simulink model "BATTERY_PV_IMPLEMENTATION"  (R2024a)
settings: Solver=VariableStepAuto  StartTime=0.0  StopTime=0.23  RelTol=1e-3
values from neighbouring files (symbols this model uses):
  a = 1.3    [TEST.m]    (also in batter_y.m = -k_omega / J)
  beta = [0.0000, 0.0306, 0.0560, 0.0772, 0.0953, 0.1113, 0.1254, 0.1382,          0.1499, 0.1607, 0.1783, 0.2134, 0.2421, 0.2669, 0.2890, 0.3091,          0.3279, 0.3456, 0.3625, 0.3789]'    [batter_y.m]
  Cdc = 278e-3    (= 0.278)    [TEST.m]    (also in batter_y.m)
  Clink = 2 * (3 / 4) * (Pnom / Fnom * 2 / Vnom_dc^2)    (= 0.325520833333)    [batter_y.m]
  fg = 60    [TEST.m]    (also in batter_y.m)
  Fnom = 60    [batter_y.m]
  Gn = 1000    [TEST.m]    (also in batter_y.m)
  Ipv_n = Isc_n*(Rp+Rs)/Rp    (= 8.21426513558)    [TEST.m]    (also in batter_y.m)
  Isc_n = 8.21    [TEST.m]    (also in batter_y.m)
  k = 1.3806503e-23    [TEST.m]    (also in batter_y.m)
  k_I = a./(b.*tau_ref)    [batter_y.m]
  k_P = 5./(b.*tau_ref)    [batter_y.m]
  KI = 0.0032    [TEST.m]    (also in batter_y.m)
  Ki_C = Rc/tau_C    (= 0.768)    [TEST.m]    (also in batter_y.m)
  Ki_DC = omega_DC^2*Cdc    [TEST.m]    (also in batter_y.m)
  Ki_Ireg = 20    [batter_y.m]
  Ki_P = 1/(Ki_pq*tau_P)    [TEST.m]    (also in batter_y.m)
  Ki_PLL = Kp_PLL/tau_PLL    [TEST.m]    (also in batter_y.m)
  Kp_C = Lc/tau_C    (= 0.020372)    [TEST.m]    (also in batter_y.m)
  Kp_DC = 2*xi_DC*omega_DC*Cdc    [TEST.m]    (also in batter_y.m)
  Kp_Ireg = 0.3    [batter_y.m]
  Kp_P = tau_C/(Ki_pq*tau_P)    [TEST.m]    (also in batter_y.m)
  Kp_PLL = xi_PLL*2*omega_PLL/Vp    [TEST.m]    (also in batter_y.m)
  KV = -0.123    [TEST.m]    (also in batter_y.m)
  KVmp = Vmp_n/Voc_n    (= 0.799392097264)    [TEST.m]    (also in batter_y.m)
  Lc = 20.372e-6    (= 2.0372e-05)    [TEST.m]    (also in batter_y.m)
  Lchoke = 0.15    [batter_y.m]
  Ltot_pu = Lxf + Lchoke    (= 0.21)    [batter_y.m]
  Lxf = TotalLeakage    (= 0.06)    [batter_y.m]
  Np = 345    [TEST.m]    (also in batter_y.m)
  Ns = 45    [TEST.m]    (also in batter_y.m)
  Ns_cell = 54    [TEST.m]    (also in batter_y.m)
  Pnom = PnomkW*1e3    (= 500000)    [TEST.m]    (also in batter_y.m = 1500000)
  q = 1.6021764e-19    [TEST.m]    (also in batter_y.m)
  Rc = 0.768e-3    (= 0.000768)    [TEST.m]    (also in batter_y.m)
  Rchoke = 0.15 / 100    (= 0.0015)    [batter_y.m]
  Rp = 425.405    [TEST.m]    (also in batter_y.m)
  Rs = 0.221    [TEST.m]    (also in batter_y.m)
  Rtot_pu = Rxf + Rchoke    (= 0.0039)    [batter_y.m]
  Rxf = TotalLeakage / 25    (= 0.0024)    [batter_y.m]
  Tn = 25    [TEST.m]    (also in batter_y.m)
  Ts = 5e-5    (= 5e-05)    [TEST.m]    (also in batter_y.m)
  Ts_Control = 5e-5    (= 5e-05)    [TEST.m]    (also in batter_y.m)
  v = [11.2600, 11.5378, 11.8156, 12.0933, 12.3711, 12.6489, 12.9267,       13.2044, 13.4822, 13.7600, 14.2600, 15.4533, 16.6467, 17.8400,       19.0333, 20.2267, 21.4200, 22.6133, 23.8067, 25.0000]'    [batter_y.m]
  Vdc = 1200    [TEST.m]    (also in batter_y.m)
  Vnom_dc = 480    [batter_y.m]
  Vnom_prim = 2400    [batter_y.m]
  Vnom_sec = 0.85 * Vnom_dc / 2 / sqrt(2) * sqrt(3)    [batter_y.m]
  Voc_n = 32.9    [TEST.m]    (also in batter_y.m)
  Vp = Ug*sqrt(2)/sqrt(3)    [TEST.m]    (also in batter_y.m)
  Zbase = Vnom_sec^2 / Pnom    [batter_y.m]
undefined symbols (not defined in the file or in its folder): D1, Delta, Ion, Lithium, para_mdl
libraries: spsSeriesRLCBranchLib x25, slpidlib x11, spsThreePhaseSeriesRLCLoadLib x9, spsThreePhaseVIMeasurementLib x7, spsSeriesRLCLoadLib x5, spsGroundLib x5, spsThreePhaseTransformerTwoWindingsLib x5, spsabctodq0Lib x4, spsControlledVoltageSourceLib x3, spsPower3phInstantaneousLib x3, spsCurrentMeasurementLib x2, spsControlledCurrentSourceLib x2
(part 1 of 3)
settings Model: Creator=Dell  LastModifiedBy=Dell

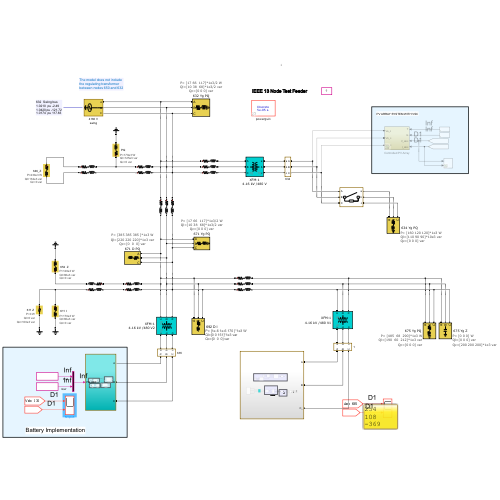
[thumbnail: Simulink's stored preview of the top-level diagram]
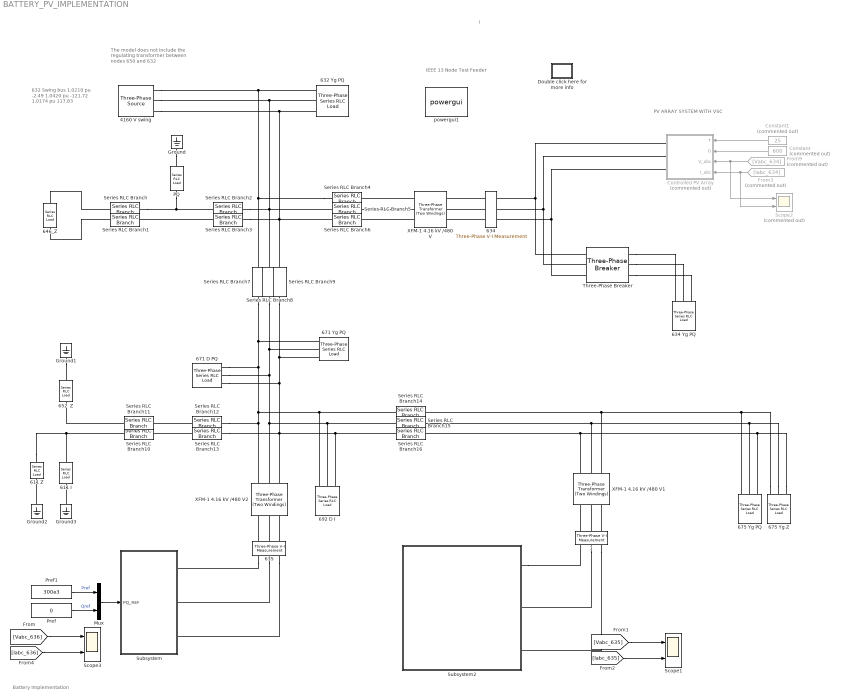
== system BATTERY_PV_IMPLEMENTATION ==
  note: Battery Implementation
  note: i
  note: PV ARRAY SYSTEM WITH VSC
  note: IEEE 13 Node Test Feeder
  note: The model does not include
      | the regulating transformer
      | between nodes 650 and 632
  note: 632 Swing bus
      | 1.0210 pu -2.49
      | 1.0420 pu -121.72
      | 1.0174 pu 117.83
  " 634 Yg PQ " : spsThreePhaseSeriesRLCLoadLib/Three-Phase Series RLC Load  LConnTagsString=A|B|C  Configuration=Y (grounded)  NominalVoltage=120e3  Vabc=[ 0.993805 1.0218 0.995862]*277.128  Vabcp=[1e3 1e3 1e3]  NominalFrequency=60  UnbalancedPower=on  ActivePower=1e+006  InductivePower=0  CapacitivePower=0  Pabc=[160 120 120]*1e3  QLabc=[110 90 90]*10e3  QCabc=[0 0 0]  Pabcp=[10e3 9e3 11e3]  QLabcp=[100 90 110]  QCabcp=[100 90 110]  Measurements=None  LoadType=constant PQ
      settings: AttributesFormatString=|
      | P= %<Pabc> W
      | Ql=%<QLabc> var
      | Qc=%<QCabc> var
  1 : spsThreePhaseVIMeasurementLib/Three-Phase V-I Measurement  VoltageMeasurement=phase-to-ground  SetLabelV=on  LabelV=Vabc_635  Vpu=off  VpuLL=off  CurrentMeasurement=yes  SetLabelI=on  LabelI=Iabc_635  Ipu=off  Pbase=100e6  Vbase=4160  OutputType=Complex  PhasorSimulation=off  PSBequivalent=0
  4160 V swing : spsThreePhaseSourceLib/Three-Phase Source  InternalConnection=Yg  VoltagePhases=on  Voltage=4.16e3  PhaseAngle=0  Voltage_phases=[ 1.021 1.042 1.0174]*2401.78  PhaseAngles_phases=[ -2.49 -121.72 117.83]  Frequency=60  NonIdealSource=off  SpecifyImpedance=on  Resistance=0.8929  Inductance=16.58e-3  ShortCircuitLevel=100e6  BaseVoltage=120e3  XRratio=10  BusType=swing  Pref=0  Qref=0  Prefabc=[0 0 0]  Qrefabc=[0 0 0]  Qmin="[-inf  -inf -inf]"  Qmax="[inf  inf inf]"
  611 I : spsSeriesRLCLoadLib/Series RLC Load  LConnTagsString=a  RConnTagsString=__new0  NominalVoltage=0.986941*2401.78  NominalFrequency=60  ActivePower=170e3  InductivePower=80e3  CapacitivePower=0  Setx0=off  InitialVoltage=0  SetiL0=off  InitialCurrent=0  Measurements=Branch voltage and current  LoadType=constant I
      settings: AttributesFormatString=|
      | P=%<ActivePower> W
      | Ql=%<InductivePower> var
      | Qc=%<CapacitivePower> var
  611 Z : spsSeriesRLCLoadLib/Series RLC Load  LConnTagsString=a  RConnTagsString=__new0  NominalVoltage=4160/sqrt(3)  NominalFrequency=60  ActivePower=0  InductivePower=0  CapacitivePower=100e3  Setx0=off  InitialVoltage=0  SetiL0=off  InitialCurrent=0  Measurements=None  LoadType=constant Z
      settings: AttributesFormatString=|
      | P=%<ActivePower> W
      | Ql=%<InductivePower> var
      | Qc=%<CapacitivePower> var
  632 Yg PQ : spsThreePhaseSeriesRLCLoadLib/Three-Phase Series RLC Load  LConnTagsString=A|B|C  Configuration=Y (grounded)  NominalVoltage=120e3  Vabc=[ 1.021 1.042 1.0174]*2401.78  Vabcp=[1e3 1e3 1e3]  NominalFrequency=60  UnbalancedPower=on  ActivePower=1e+006  InductivePower=0  CapacitivePower=0  Pabc="[17 66  117]*1e3/2"  QLabc="[10 38  68]*1e3/2"  QCabc=[0 0 0]  Pabcp=[10e3 9e3 11e3]  QLabcp=[100 90 110]  QCabcp=[100 90 110]  Measurements=None  LoadType=constant PQ
      settings: AttributesFormatString=|
      | P= %<Pabc> W
      | Ql=%<QLabc> var
      | Qc=%<QCabc> var
  634 : spsThreePhaseVIMeasurementLib/Three-Phase V-I Measurement  VoltageMeasurement=phase-to-ground  SetLabelV=on  LabelV=Vabc_634  Vpu=off  VpuLL=off  CurrentMeasurement=yes  SetLabelI=on  LabelI=Iabc_634  Ipu=off  Pbase=100e6  Vbase=4160  OutputType=Complex  PhasorSimulation=off  PSBequivalent=0
  635 : spsThreePhaseVIMeasurementLib/Three-Phase V-I Measurement  VoltageMeasurement=phase-to-ground  SetLabelV=on  LabelV=Vabc_636  Vpu=off  VpuLL=off  CurrentMeasurement=yes  SetLabelI=on  LabelI=Iabc_636  Ipu=off  Pbase=100e6  Vbase=4160  OutputType=Complex  PhasorSimulation=off  PSBequivalent=0
  646_Z : spsSeriesRLCLoadLib/Series RLC Load  LConnTagsString=a  RConnTagsString=__new0  NominalVoltage=4160  NominalFrequency=60  ActivePower=230e3  InductivePower=132e3  CapacitivePower=0  Setx0=off  InitialVoltage=0  SetiL0=off  InitialCurrent=0  Measurements=None  LoadType=constant Z
      settings: AttributesFormatString=|
      | P=%<ActivePower> W
      | Ql=%<InductivePower> var
      | Qc=%<CapacitivePower> var
  "652  Z " : spsSeriesRLCLoadLib/Series RLC Load  LConnTagsString=a  RConnTagsString=__new0  NominalVoltage=4160/sqrt(3)  NominalFrequency=60  ActivePower=128e3  InductivePower=86e3  CapacitivePower=0  Setx0=off  InitialVoltage=0  SetiL0=off  InitialCurrent=0  Measurements=None  LoadType=constant Z
      settings: AttributesFormatString=|
      | P=%<ActivePower> W
      | Ql=%<InductivePower> var
      | Qc=%<CapacitivePower> var
  671 D PQ : spsThreePhaseSeriesRLCLoadLib/Three-Phase Series RLC Load  LConnTagsString=A|B|C  Configuration=Delta  NominalVoltage=120e3  Vabc="[1  1  1]*120e3/sqrt(3)"  Vabcp=[ 1.73773 1.77224 1.71484]*2401.78  NominalFrequency=60  UnbalancedPower=on  ActivePower=1e+006  InductivePower=0  CapacitivePower=0  Pabc="[17 66  117]*1e3/2"  QLabc="[10 38  68]*1e3/2"  QCabc=[0 0 0]  Pabcp=[385 385 385 ]*1e3  QLabcp=[220 220 220]*1e3  QCabcp="[0  0  0]"  Measurements=Branch voltages and currents  LoadType=constant PQ
      settings: AttributesFormatString=|
      | P= %<Pabcp> W
      | Ql=%<QLabcp> var
      | Qc=%<QCabcp> var
  671 Yg PQ : spsThreePhaseSeriesRLCLoadLib/Three-Phase Series RLC Load  LConnTagsString=A|B|C  Configuration=Y (grounded)  NominalVoltage=120e3  Vabc=[ 0.987076 1.0519 0.978043]*2401.78  Vabcp=[1e3 1e3 1e3]  NominalFrequency=60  UnbalancedPower=on  ActivePower=1e+006  InductivePower=0  CapacitivePower=0  Pabc="[17 66  117]*1e3/2"  QLabc="[10 38  68]*1e3/2"  QCabc=[0 0 0]  Pabcp=[10e3 9e3 11e3]  QLabcp=[100 90 110]  QCabcp=[100 90 110]  Measurements=None  LoadType=constant PQ
      settings: AttributesFormatString=|
      | P= %<Pabc> W
      | Ql=%<QLabc> var
      | Qc=%<QCabc> var
  675 Yg PQ : spsThreePhaseSeriesRLCLoadLib/Three-Phase Series RLC Load  LConnTagsString=A|B|C  Configuration=Y (grounded)  NominalVoltage=120e3  Vabc=[ 0.98063 1.05431 0.975983]*2401.78  Vabcp=[1e3 1e3 1e3]  NominalFrequency=60  UnbalancedPower=on  ActivePower=1e+006  InductivePower=0  CapacitivePower=0  Pabc="[485  68  290]*1e3"  QLabc="[190  60  212]*1e3"  QCabc=[0 0 0]  Pabcp=[10e3 9e3 11e3]  QLabcp=[100 90 110]  QCabcp=[100 90 110]  Measurements=Branch voltages and currents  LoadType=constant PQ
      settings: AttributesFormatString=|
      | P= %<Pabc> W
      | Ql=%<QLabc> var
      | Qc=%<QCabc> var
  675 Yg Z : spsThreePhaseSeriesRLCLoadLib/Three-Phase Series RLC Load  LConnTagsString=A|B|C  Configuration=Y (grounded)  NominalVoltage=120e3  Vabc="[1  1  1]*4160/sqrt(3)"  Vabcp=[1e3 1e3 1e3]  NominalFrequency=60  UnbalancedPower=on  ActivePower=1e+006  InductivePower=0  CapacitivePower=0  Pabc=[0 0 0]  QLabc=[0 0 0]  QCabc=[200 200 200]*1e3  Pabcp=[10e3 9e3 11e3]  QLabcp=[100 90 110]  QCabcp=[100 90 110]  Measurements=None  LoadType=constant Z
      settings: AttributesFormatString=|
      | P= %<Pabc> W
      | Ql=%<QLabc> var
      | Qc=%<QCabc> var
  692 D I : spsThreePhaseSeriesRLCLoadLib/Three-Phase Series RLC Load  LConnTagsString=A|B|C  Configuration=Delta  NominalVoltage=120e3  Vabc="[1  1  1]*120e3/sqrt(3)"  Vabcp=[ 1.73488 1.75203 1.72341]*2401.78  NominalFrequency=60  UnbalancedPower=on  ActivePower=1e+006  InductivePower=0  CapacitivePower=0  Pabc="[17 66  117]*1e3/2"  QLabc="[10 38  68]*1e3/2"  QCabc=[0 0 0]  Pabcp=[1e-6 1e-6 170 ]*1e3  QLabcp=[0 0 151]*1e3  QCabcp="[0  0  0]"  Measurements=Branch voltages and currents  LoadType=constant I
      settings: AttributesFormatString=|
      | P= %<Pabcp> W
      | Ql=%<QLabcp> var
      | Qc=%<QCabcp> var
  Constant : Constant  Commented=on  Value=600
  Constant1 : Constant  Commented=on  Value=25
  Controlled PV Array : Subsystem  Commented=on
      settings: PortSchema="{\"entries\":[{\"content\":{\"sides\":[{\"content\":{\"connectorIds\":[\"LConn1\",\"LConn2\",\"LConn3\"]},\"type\":\"ConnectorPlacement.EquallySpacedRectSide\",\"uuid\":\"92a05cf9-a19b-475d-bffb-9406018f82f4\"},{\"content\":{\"connectorIds\":[\"In1\",\"In2\",\"In3\",\"In4\"],\"side\":\"RIGHT\"},\"type\":\"ConnectorPlacement.EquallySpacedRectSide\",\"uuid\":\"83076eb6-0a86-49d7-8932-035501cdc6f6\"},{\"content\":{\"side\":\"TOP\"},\"type\":\"ConnectorPlacement.EquallySpacedRectSide\",\"uuid\":\"ba2310df-ee07-4a5c-88ff-ef0f81658322\"}]},\"type\":\"ConnectorPlacement.EquallySpacedConnector\",\"uuid\":\"9e64c472-0dae-4bb4-8eb3-3329c328d412\"}],\"packageUris\":[\"http://schema.mathworks.com/mf0/Connector/R2020b\"],\"version\":\"1.0\"}"
  Double click here for more info : Subsystem
      settings: OpenFcn=showdemo(bdroot(gcb))
      mask Display: disp('?')
  From3 : From  Commented=on  GotoTag=Iabc_634  TagVisibility=global
  From9 : From  Commented=on  GotoTag=Vabc_634  TagVisibility=global
  Ground{,1..3} (4 alike) : spsGroundLib/Ground  LConnTagsString=a
  Mux : Mux  Inputs=2
  PQ : spsSeriesRLCLoadLib/Series RLC Load  LConnTagsString=a  RConnTagsString=__new0  NominalVoltage=1.03289*2401.78  NominalFrequency=60  ActivePower=170e3  InductivePower=125e3  CapacitivePower=0  Setx0=off  InitialVoltage=0  SetiL0=off  InitialCurrent=0  Measurements=None  LoadType=constant PQ
      settings: AttributesFormatString=|
      | P=%<ActivePower> W
      | Ql=%<InductivePower> var
      | Qc=%<CapacitivePower> var
  Pref : Constant  Value=0
  Pref1 : Constant  Value=300e3
  Scope1 : Scope  NumInputPorts=2
  Scope2 : Scope  Commented=on  NumInputPorts=2
  Scope3 : Scope  NumInputPorts=2
  Series RLC Branch : spsSeriesRLCBranchLib/Series RLC Branch  LConnTagsString=__new0  RConnTagsString=__new0  BranchType=RL  Resistance=0.07553  Inductance=0.20302e-3  SetiL0=off  InitialCurrent=0  Capacitance=1e-6  Setx0=off  InitialVoltage=0  Measurements=None
  Series RLC Branch1 : spsSeriesRLCBranchLib/Series RLC Branch  LConnTagsString=__new0  RConnTagsString=__new0  BranchType=RL  Resistance=0.07553  Inductance=0.20302e-3  SetiL0=off  InitialCurrent=0  Capacitance=1e-6  Setx0=off  InitialVoltage=0  Measurements=None
  Series RLC Branch10 : spsSeriesRLCBranchLib/Series RLC Branch  LConnTagsString=__new0  RConnTagsString=__new0  BranchType=RL  Resistance=0.07552  Inductance=0.20308e-3  SetiL0=off  InitialCurrent=0  Capacitance=1e-6  Setx0=off  InitialVoltage=0  Measurements=None
  Series RLC Branch11 : spsSeriesRLCBranchLib/Series RLC Branch  LConnTagsString=__new0  RConnTagsString=__new0  BranchType=RL  Resistance=0.20340  Inductance=0.20593e-3  SetiL0=off  InitialCurrent=0  Capacitance=1e-6  Setx0=off  InitialVoltage=0  Measurements=None
  Series RLC Branch12 : spsSeriesRLCBranchLib/Series RLC Branch  LConnTagsString=__new0  RConnTagsString=__new0  BranchType=RL  Resistance=0.07521  Inductance=0.20450e-3  SetiL0=off  InitialCurrent=0  Capacitance=1e-6  Setx0=off  InitialVoltage=0  Measurements=None
  Series RLC Branch13 : spsSeriesRLCBranchLib/Series RLC Branch  LConnTagsString=__new0  RConnTagsString=__new0  BranchType=RL  Resistance=0.07521  Inductance=0.20450e-3  SetiL0=off  InitialCurrent=0  Capacitance=1e-6  Setx0=off  InitialVoltage=0  Measurements=None
  Series RLC Branch14 : spsSeriesRLCBranchLib/Series RLC Branch  LConnTagsString=__new0  RConnTagsString=__new0  BranchType=RL  Resistance=0.07559  Inductance=0.11210e-3  SetiL0=off  InitialCurrent=0  Capacitance=1e-6  Setx0=off  InitialVoltage=0  Measurements=None
  Series RLC Branch15 : spsSeriesRLCBranchLib/Series RLC Branch  LConnTagsString=__new0  RConnTagsString=__new0  BranchType=RL  Resistance=0.07559  Inductance=0.11210e-3  SetiL0=off  InitialCurrent=0  Capacitance=1e-6  Setx0=off  InitialVoltage=0  Measurements=None
  Series RLC Branch16 : spsSeriesRLCBranchLib/Series RLC Branch  LConnTagsString=__new0  RConnTagsString=__new0  BranchType=RL  Resistance=0.07559  Inductance=0.11210e-3  SetiL0=off  InitialCurrent=0  Capacitance=1e-6  Setx0=off  InitialVoltage=0  Measurements=None
  Series RLC Branch2 : spsSeriesRLCBranchLib/Series RLC Branch  LConnTagsString=__new0  RConnTagsString=__new0  BranchType=RL  Resistance=0.12589  Inductance=0.33837e-3  SetiL0=off  InitialCurrent=0  Capacitance=1e-6  Setx0=off  InitialVoltage=0  Measurements=None
  Series RLC Branch3 : spsSeriesRLCBranchLib/Series RLC Branch  LConnTagsString=__new0  RConnTagsString=__new0  BranchType=RL  Resistance=0.12589  Inductance=0.33837e-3  SetiL0=off  InitialCurrent=0  Capacitance=1e-6  Setx0=off  InitialVoltage=0  Measurements=None
  Series RLC Branch4 : spsSeriesRLCBranchLib/Series RLC Branch  LConnTagsString=__new0  RConnTagsString=__new0  BranchType=RL  Resistance=0.07126  Inductance=0.29675e-3  SetiL0=off  InitialCurrent=0  Capacitance=1e-6  Setx0=off  InitialVoltage=0  Measurements=None
  Series RLC Branch5 : spsSeriesRLCBranchLib/Series RLC Branch  LConnTagsString=__new0  RConnTagsString=__new0  BranchType=RL  Resistance=0.07126  Inductance=0.29675e-3  SetiL0=off  InitialCurrent=0  Capacitance=1e-6  Setx0=off  InitialVoltage=0  Measurements=None
  Series RLC Branch6 : spsSeriesRLCBranchLib/Series RLC Branch  LConnTagsString=__new0  RConnTagsString=__new0  BranchType=RL  Resistance=0.07126  Inductance=0.29675e-3  SetiL0=off  InitialCurrent=0  Capacitance=1e-6  Setx0=off  InitialVoltage=0  Measurements=None
  Series RLC Branch7 : spsSeriesRLCBranchLib/Series RLC Branch  LConnTagsString=__new0  RConnTagsString=__new0  BranchType=RL  Resistance=0.13124  Inductance=1.03632e-3  SetiL0=off  InitialCurrent=0  Capacitance=1e-6  Setx0=off  InitialVoltage=0  Measurements=None
  Series RLC Branch8 : spsSeriesRLCBranchLib/Series RLC Branch  LConnTagsString=__new0  RConnTagsString=__new0  BranchType=RL  Resistance=0.13124  Inductance=1.03632e-3  SetiL0=off  InitialCurrent=0  Capacitance=1e-6  Setx0=off  InitialVoltage=0  Measurements=None
  Series RLC Branch9 : spsSeriesRLCBranchLib/Series RLC Branch  LConnTagsString=__new0  RConnTagsString=__new0  BranchType=RL  Resistance=0.13124  Inductance=1.03632e-3  SetiL0=off  InitialCurrent=0  Capacitance=1e-6  Setx0=off  InitialVoltage=0  Measurements=None
  Subsystem : Subsystem
  Subsystem2 : Subsystem
  Three-Phase Breaker : spsThreePhaseBreakerLib/Three-Phase Breaker  InitialState=open  SwitchA=on  SwitchB=on  SwitchC=on  SwitchTimes=0.3  External=off  BreakerResistance=0.01  SnubberResistance=1e6  SnubberCapacitance=inf  Measurements=None
  XFM-1 4.16 kV /480 V : spsThreePhaseTransformerTwoWindingsLib/Three-Phase Transformer (Two Windings)  Winding1Connection=Yg  Winding2Connection=Yg  CoreType=Three single-phase transformers  SetSaturation=off  Hysteresis=off  DataFile='hysteresis'  SetInitialFlux=off  Measurements=None  UNITS=pu  NominalPower=[ 500e3 , 60 ]  Winding1=[4160 0.011 0.02]  Winding2=[480 0 0]  Rm=500  Lm=500  L0=0.5  Saturation=[0 0;0.0024 1.2;1 1.52]  InitialFluxes=[0.8 -0.8 0.7]  BreakLoop=off  DiscreteSolver=Trapezoidal iterative  DataType=off  TransfoNumber=1
  XFM-1 4.16 kV /480 V1 : spsThreePhaseTransformerTwoWindingsLib/Three-Phase Transformer (Two Windings)  Winding1Connection=Yg  Winding2Connection=Yg  CoreType=Three single-phase transformers  SetSaturation=off  Hysteresis=off  DataFile='hysteresis'  SetInitialFlux=off  Measurements=None  UNITS=pu  NominalPower=[ 500e3 , 60 ]  Winding1=[4160 0.011 0.02]  Winding2=[480 0 0]  Rm=500  Lm=500  L0=0.5  Saturation=[0 0;0.0024 1.2;1 1.52]  InitialFluxes=[0.8 -0.8 0.7]  BreakLoop=off  DiscreteSolver=Trapezoidal iterative  DataType=off  TransfoNumber=1
  XFM-1 4.16 kV /480 V2 : spsThreePhaseTransformerTwoWindingsLib/Three-Phase Transformer (Two Windings)  Winding1Connection=Yg  Winding2Connection=Yg  CoreType=Three single-phase transformers  SetSaturation=off  Hysteresis=off  DataFile='hysteresis'  SetInitialFlux=off  Measurements=None  UNITS=pu  NominalPower=[ 500e3 , 60 ]  Winding1=[4160 0.011 0.02]  Winding2=[480 0 0]  Rm=500  Lm=500  L0=0.5  Saturation=[0 0;0.0024 1.2;1 1.52]  InitialFluxes=[0.8 -0.8 0.7]  BreakLoop=off  DiscreteSolver=Trapezoidal iterative  DataType=off  TransfoNumber=1
  powergui1 : spspowerguiLib/powergui  Priority=1  SimulationMode=Discrete  SampleTime=5e-5  frequency=60  Iterations=50  frequencyindice=0  Pbase=100e3  ErrMax=0.0001  UnitsV=kV  UnitsW=kW  buscounter=0  FunctionMessages=off  echomessages=off  EnableUseOfTLC=off  CurrentSourceSwitches=off  DisableSnubberDevices=off  DisableRonSwitches=off  DisableVfSwitches=off  DisplayEquations=off  AutomaticDiscreteSolvers=off  SolverType=Tustin/Backward Euler (TBE)  Interpol=off  ExternalGateDelay=off  methode=off  Ts=0  x0status=blocks  SPID=off  SwTol=0  HookPort=off  NonlinearTolerance=1e-4  nMaxIteration=100  ContinueOnMaxIteration=off  RestoreLinks=warning  ResistiveCurrentMeasurement=off  Frange=[0:2:500]  Ylog=off  Xlog=on  ShowGrid=off  save=off  variable=ZData  structure=0  ZoomFFT=on  StartTime=0.0  cycles=1  DisplayStyle=1  fundamental=60  FreqAxis=off  MaxFrequency=1000  frequencyindicesteady=1  RmsSteady=1  display=off
  wires:
  From3/1 -> Scope2/2, Controlled PV Array/4(I_abc)
  [Iabc_636] -> Scope3/2
  [Vabc_636] -> Scope3/1
  Constant/1 -> Controlled PV Array/2(G)
  From9/1 -> Scope2/1, Controlled PV Array/3(V_abc)
  Constant1/1 -> Controlled PV Array/1(T)
  Pref1/1 -> Mux/1  "Pref"
  Pref/1 -> Mux/2  "Qref"
  Mux/1 -> Subsystem/1(PQ_REF)
  [Vabc_635] -> Scope1/1
  [Iabc_635] -> Scope1/2
  connections:
  Series RLC Branch13/RConn1 -- 671 D PQ/LConn3 -- Series RLC Branch9/RConn1 -- 671 Yg PQ/LConn3 -- XFM-1 4.16 kV /480 V2/LConn1 -- 692 D I/LConn3 -- Series RLC Branch16/LConn1
  634/LConn1 -- Controlled PV Array/LConn1 -- Three-Phase Breaker/LConn1
  Series RLC Branch4/LConn1 -- Series RLC Branch7/LConn1 -- 632 Yg PQ/LConn1 -- 4160 V swing/RConn1
  Series RLC Branch/RConn1 -- PQ/LConn1 -- Series RLC Branch2/LConn1
  671 D PQ/LConn2 -- 692 D I/LConn2 -- Series RLC Branch15/LConn1 -- XFM-1 4.16 kV /480 V2/LConn2 -- Series RLC Branch8/RConn1 -- 671 Yg PQ/LConn2
  611 Z/LConn1 -- 611 I/LConn1 -- Series RLC Branch10/LConn1
  Series RLC Branch12/RConn1 -- XFM-1 4.16 kV /480 V2/LConn3 -- 692 D I/LConn1 -- Series RLC Branch14/LConn1 -- 671 D PQ/LConn1 -- Series RLC Branch7/RConn1 -- 671 Yg PQ/LConn1
  Series RLC Branch2/RConn1 -- 632 Yg PQ/LConn2 -- 4160 V swing/RConn2 -- Series RLC Branch8/LConn1 -- Series RLC Branch5/LConn1
  Series RLC Branch3/RConn1 -- 632 Yg PQ/LConn3 -- 4160 V swing/RConn3 -- Series RLC Branch9/LConn1 -- Series RLC Branch6/LConn1
  634/LConn3 -- Controlled PV Array/LConn3 -- Three-Phase Breaker/LConn3
  634/LConn2 -- Controlled PV Array/LConn2 -- Three-Phase Breaker/LConn2
  675 Yg Z/LConn1 -- Series RLC Branch14/RConn1 -- XFM-1 4.16 kV /480 V1/LConn1 -- 675 Yg PQ/LConn1
  675 Yg Z/LConn3 -- XFM-1 4.16 kV /480 V1/LConn3 -- Series RLC Branch16/RConn1 -- 675 Yg PQ/LConn3
  675 Yg Z/LConn2 -- Series RLC Branch15/RConn1 -- XFM-1 4.16 kV /480 V1/LConn2 -- 675 Yg PQ/LConn2
  635/RConn1 -- XFM-1 4.16 kV /480 V2/RConn3
  XFM-1 4.16 kV /480 V/LConn3 -- Series RLC Branch6/RConn1
  Series RLC Branch12/LConn1 -- Series RLC Branch11/LConn1
  Three-Phase Breaker/RConn1 -- " 634 Yg PQ "/LConn1
  Ground1/LConn1 -- "652  Z "/RConn1
  635/RConn2 -- XFM-1 4.16 kV /480 V2/RConn2
  635/RConn3 -- XFM-1 4.16 kV /480 V2/RConn1
  634/RConn1 -- XFM-1 4.16 kV /480 V/RConn1
  634/RConn2 -- XFM-1 4.16 kV /480 V/RConn2
  634/RConn3 -- XFM-1 4.16 kV /480 V/RConn3
  Series RLC Branch3/LConn1 -- Series RLC Branch1/RConn1
  Series RLC Branch11/RConn1 -- "652  Z "/LConn1
  Three-Phase Breaker/RConn2 -- " 634 Yg PQ "/LConn2
  Series RLC Branch5/RConn1 -- XFM-1 4.16 kV /480 V/LConn2
  XFM-1 4.16 kV /480 V/LConn1 -- Series RLC Branch4/RConn1
  Ground3/LConn1 -- 611 I/RConn1
  Ground2/LConn1 -- 611 Z/RConn1
  Three-Phase Breaker/RConn3 -- " 634 Yg PQ "/LConn3
  Series RLC Branch/LConn1 -- 646_Z/LConn1
  Ground/LConn1 -- PQ/RConn1
  Series RLC Branch1/LConn1 -- 646_Z/RConn1
  Series RLC Branch13/LConn1 -- Series RLC Branch10/RConn1
  635/LConn1 -- Subsystem/RConn1
  635/LConn2 -- Subsystem/RConn2
  635/LConn3 -- Subsystem/RConn3
  1/LConn3 -- Subsystem2/RConn3
  Subsystem2/RConn1 -- 1/LConn1
  1/LConn2 -- Subsystem2/RConn2
  1/RConn3 -- XFM-1 4.16 kV /480 V1/RConn1
  1/RConn2 -- XFM-1 4.16 kV /480 V1/RConn2
  1/RConn1 -- XFM-1 4.16 kV /480 V1/RConn3

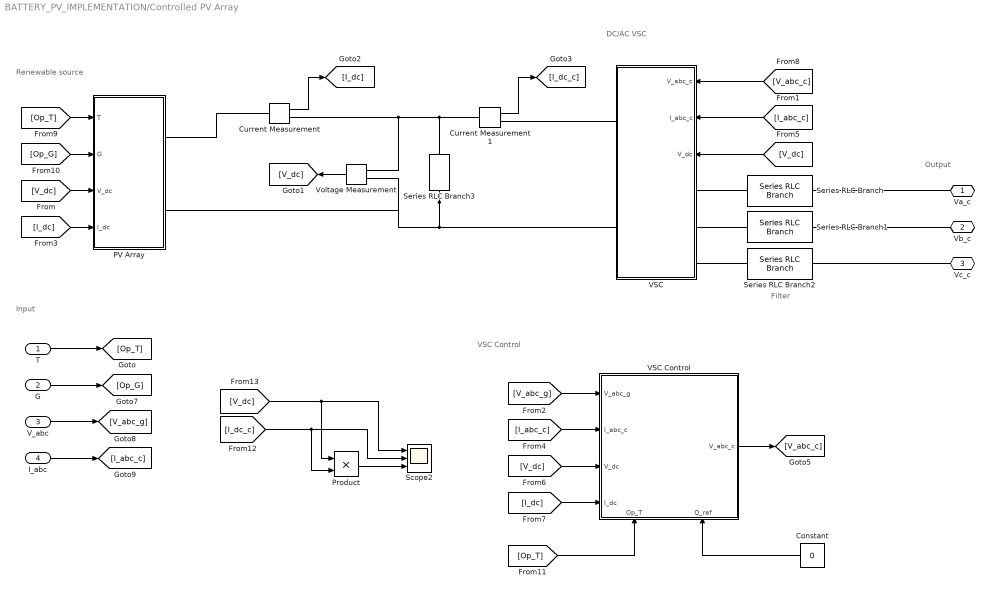
== system BATTERY_PV_IMPLEMENTATION/Controlled PV Array ==
  note: Output
  note: Input
  note: Filter
  note: Renewable source
  note: VSC Control
  note: DC/AC VSC
  T : Inport
  G : Inport  Port=2
  V_abc : Inport  Port=3
  I_abc : Inport  Port=4
  Constant : Constant  Value=0
  Current Measurement : spsCurrentMeasurementLib/Current Measurement  PhasorSimulation=off  OutputType=Complex  PSBequivalent=0
  Current Measurement1 : spsCurrentMeasurementLib/Current Measurement  PhasorSimulation=off  OutputType=Complex  PSBequivalent=0
  PV Array : Subsystem
  Product : Product
  Scope2 : Scope  NumInputPorts=3
  Series RLC Branch : spsSeriesRLCBranchLib/Series RLC Branch  LConnTagsString=__new0  RConnTagsString=__new0  BranchType=RL  Resistance=Rc  Inductance=Lc  SetiL0=off  InitialCurrent=0  Capacitance=1e-6  Setx0=off  InitialVoltage=0  Measurements=None
  Series RLC Branch1 : spsSeriesRLCBranchLib/Series RLC Branch  LConnTagsString=__new0  RConnTagsString=__new0  BranchType=RL  Resistance=Rc  Inductance=Lc  SetiL0=off  InitialCurrent=0  Capacitance=1e-6  Setx0=off  InitialVoltage=0  Measurements=None
  Series RLC Branch2 : spsSeriesRLCBranchLib/Series RLC Branch  LConnTagsString=__new0  RConnTagsString=__new0  BranchType=RL  Resistance=Rc  Inductance=Lc  SetiL0=off  InitialCurrent=0  Capacitance=1e-6  Setx0=off  InitialVoltage=0  Measurements=None
  Series RLC Branch3 : spsSeriesRLCBranchLib/Series RLC Branch  LConnTagsString=__new0  RConnTagsString=__new0  BranchType=C  Resistance=0.3  Inductance=1e-3  SetiL0=off  InitialCurrent=0  Capacitance=Cdc  Setx0=on  InitialVoltage=Vdc  Measurements=None
  VSC : Subsystem
  VSC Control : Subsystem
      settings: PortSchema="{\"entries\":[{\"content\":{\"sides\":[{\"content\":{\"connectorIds\":[\"In1\",\"In2\",\"In3\",\"In4\"]},\"type\":\"ConnectorPlacement.EquallySpacedRectSide\",\"uuid\":\"1f0c866f-1355-4493-8a8b-fecd52da2e06\"},{\"content\":{\"connectorIds\":[\"Out1\"],\"side\":\"RIGHT\"},\"type\":\"ConnectorPlacement.EquallySpacedRectSide\",\"uuid\":\"e0482316-46fe-491c-835b-46d73fa6817a\"},{\"content\":{\"side\":\"TOP\"},\"type\":\"ConnectorPlacement.EquallySpacedRectSide\",\"uuid\":\"b85aba4d-c629-42a9-b30e-3179992b26cb\"},{\"content\":{\"connectorIds\":[\"In5\",\"In6\"],\"side\":\"BOTTOM\"},\"type\":\"ConnectorPlacement.EquallySpacedRectSide\",\"uuid\":\"2c79aeba-fb98-4b17-8331-d72a75796cf8\"}]},\"type\":\"ConnectorPlacement.EquallySpacedConnector\",\"uuid\":\"5586ce08-6872-4275-b1b0-323c6fc0897a\"}],\"packageUris\":[\"http://schema.mathworks.com/mf0/Connector/R2020b\"],\"version\":\"1.0\"}"
  Voltage Measurement : spsVoltageMeasurementLib/Voltage Measurement  PhasorSimulation=off  OutputType=Complex  PSBequivalent=0
  Va_c : PMIOPort  Side=Left
  Vb_c : PMIOPort  Port=2  Side=Left
  Vc_c : PMIOPort  Port=3  Side=Left
  wires:
  [V_abc_c] -> VSC/1(V_abc_c)
  Constant/1 -> VSC Control/6(Q_ref)
  I_abc/1 -> [I_abc_c]
  Current Measurement1/1 -> [I_dc_c]
  [V_dc] -> Scope2/1, Product/1
  [I_dc_c] -> Scope2/2, Product/2
  [I_dc] -> VSC Control/4(I_dc)
  Voltage Measurement/1 -> [V_dc]
  [V_abc_g] -> VSC Control/1(V_abc_g)
  VSC Control/1(V_abc_c) -> [V_abc_c]
  [V_dc] -> PV Array/3(V_dc)
  Current Measurement/1 -> [I_dc]
  Product/1 -> Scope2/3
  [Op_T] -> VSC Control/5(Op_T)
  [V_dc] -> VSC/3(V_dc)
  V_abc/1 -> [V_abc_g]
  [Op_T] -> PV Array/1(T)
  [V_dc] -> VSC Control/3(V_dc)
  [Op_G] -> PV Array/2(G)
  [I_abc_c] -> VSC Control/2(I_abc_c)
  [I_abc_c] -> VSC/2(I_abc_c)
  [I_dc] -> PV Array/4(I_dc)
  G/1 -> [Op_G]
  T/1 -> [Op_T]
  connections:
  VSC/LConn2 -- Series RLC Branch1/RConn1
  Series RLC Branch3/RConn1 -- Voltage Measurement/LConn2 -- PV Array/RConn2 -- VSC/RConn2
  Current Measurement1/LConn1 -- Series RLC Branch3/LConn1 -- Current Measurement/RConn1 -- Voltage Measurement/LConn1
  PV Array/RConn1 -- Current Measurement/LConn1
  VSC/LConn1 -- Series RLC Branch/RConn1
  VSC/LConn3 -- Series RLC Branch2/RConn1
  Va_c/RConn1 -- Series RLC Branch/LConn1
  VSC/RConn1 -- Current Measurement1/RConn1
  Vc_c/RConn1 -- Series RLC Branch2/LConn1
  Vb_c/RConn1 -- Series RLC Branch1/LConn1

== system BATTERY_PV_IMPLEMENTATION/Double click here for more info ==

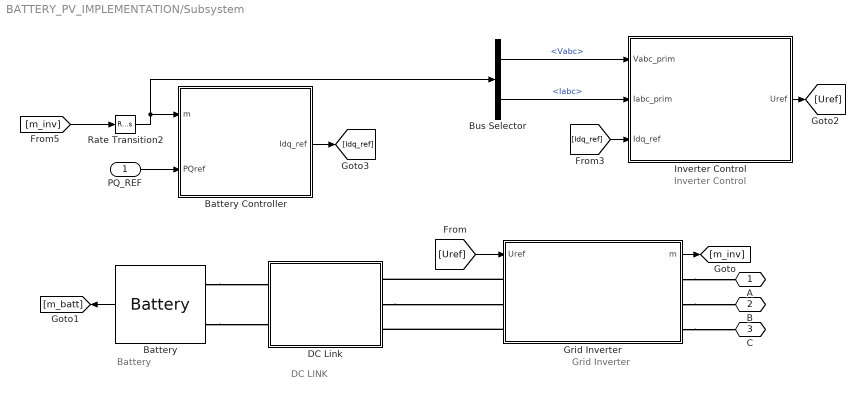
== system BATTERY_PV_IMPLEMENTATION/Subsystem ==
  note: Inverter Control
  note: Grid Inverter
  note: DC LINK
  note: Battery
  PQ_REF : Inport
  Battery : spsBatteryLib/Battery  BatType=Lithium-Ion  ShowTempParam=off  ThermalPreset=no  ShowAgeParam=off  NomV=Vnom_dc  NomQ=Bcap  SOC=75  Batt_Tr=30  PresetModel=on  MaxQ=500  MinV=360  FullV=558.7138  Dis_rate=217.3913  R=0.0096  Normal_OP=452.1739  expZone="[518.5852      24.56522]"  current=[6.5 13 32.5]  Units=Time  Tci=20  NomT=25  T2=0  MaxQ2=2.208  FullV2=3.45  Normal_OP2=2.8  expZone2="[3.22        0.23]"  Rca=0.6  ti=1000  Dp=0  Neq0=0  Tsim=1e6  Ta1=25  Qeol=5.4*0.9  Reol=0.013333*1.2  Char_age=[2.3478, 3]  Dis_age=[2.3478, 10]  N1=1500  N2=10500  N3=1000  N4=1400  Ta2=45  N5=950
      settings: LibrarySourceBlock=electricdrivelib/Extra Sources/Battery
  Battery Controller : Subsystem  SystemSampleTime=Ts
  Bus Selector : BusSelector  OutputSignals=Vabc,Iabc
  DC Link : Subsystem
  Grid Inverter : Subsystem
  Inverter Control : Subsystem
  Rate Transition2 : RateTransition  OutPortSampleTime=5e-5
  A : PMIOPort  Side=Right
  B : PMIOPort  Port=2  Side=Right
  C : PMIOPort  Port=3  Side=Right
  wires:
  Grid Inverter/1(m) -> [m_inv]
  [m_inv] -> Rate Transition2/1
  Bus Selector/2 -> Inverter Control/2(Iabc_prim)  "<Iabc>"
  Bus Selector/1 -> Inverter Control/1(Vabc_prim)  "<Vabc>"
  Rate Transition2/1 -> Battery Controller/1(m), Bus Selector/1
  Battery/1 -> [m_batt]
  PQ_REF/1 -> Battery Controller/2(PQref)
  [Uref] -> Grid Inverter/1(Uref)
  Inverter Control/1(Uref) -> [Uref]
  Battery Controller/1(Idq_ref) -> [Idq_ref]
  [Idq_ref] -> Inverter Control/3(Idq_ref)
  connections:
  Grid Inverter/LConn1 -- DC Link/RConn1
  Grid Inverter/LConn3 -- DC Link/RConn3
  DC Link/RConn2 -- Grid Inverter/LConn2
  Grid Inverter/RConn1 -- A/RConn1
  Battery/LConn2 -- DC Link/LConn2
  Battery/LConn1 -- DC Link/LConn1
  Grid Inverter/RConn2 -- B/RConn1
  Grid Inverter/RConn3 -- C/RConn1

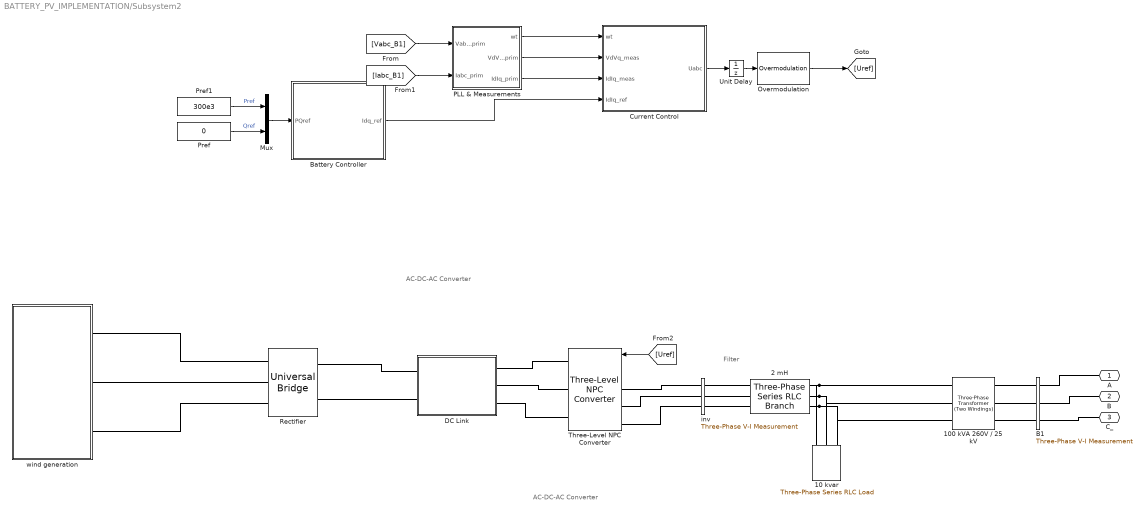
== system BATTERY_PV_IMPLEMENTATION/Subsystem2 ==
  note: AC-DC-AC Converter
  note: AC-DC-AC Converter
  note: Filter
  10 kvar : spsThreePhaseSeriesRLCLoadLib/Three-Phase Series RLC Load  LConnTagsString=A|B|C  Configuration=Delta  NominalVoltage=Vnom_sec  Vabc=[1e3 1e3 1e3]  Vabcp=[1e3 1e3 1e3]  NominalFrequency=Fnom  UnbalancedPower=off  ActivePower=Pc  InductivePower=0  CapacitivePower=Qc  Pabc=[10e3 9e3 11e3]  QLabc=[100 90 110]  QCabc=[100 90 110]  Pabcp=[10e3 9e3 11e3]  QLabcp=[100 90 110]  QCabcp=[100 90 110]  Measurements=None  LoadType=constant Z
  100 kVA 260V / 25 kV : spsThreePhaseTransformerTwoWindingsLib/Three-Phase Transformer (Two Windings)  Winding1Connection=Yg  Winding2Connection=Delta (D1)  CoreType=Three single-phase transformers  SetSaturation=off  Hysteresis=off  DataFile='hysteresis'  SetInitialFlux=off  Measurements=None  UNITS=pu  NominalPower=[Pnom Fnom ]  Winding1=[ Vnom_prim , Rxf/2 , Lxf/2 ]  Winding2=[ Vnom_sec , Rxf/2 , Lxf/2 ]  Rm=200  Lm=200  L0=0.5  Saturation=[ 0,0 ; 0.0024,1.2 ; 1.0,1.52 ]  InitialFluxes=[ 0.8 , -0.8 , 0.7 ]  BreakLoop=off  DiscreteSolver=Trapezoidal iterative  DataType=off  TransfoNumber=0
  "2 mH " : spsThreePhaseSeriesRLCBranchLib/Three-Phase Series RLC Branch  LConnTagsString=A|B|C  RConnTagsString=A|B|C  BranchType=L  Resistance=0  Inductance=2e-3  Capacitance=inf  Measurements=None
  B1 : spsThreePhaseVIMeasurementLib/Three-Phase V-I Measurement  VoltageMeasurement=phase-to-ground  SetLabelV=on  LabelV=Vabc_B1  Vpu=off  VpuLL=off  CurrentMeasurement=yes  SetLabelI=on  LabelI=Iabc_B1  Ipu=off  Pbase=100e6  Vbase=500e3  OutputType=Magnitude  PhasorSimulation=off  PSBequivalent=0
  Battery Controller : Subsystem  SystemSampleTime=Ts
  Current Control : Subsystem  TreatAsAtomicUnit=on
  DC Link : Subsystem
  Mux : Mux  Inputs=2
  Overmodulation : spsOvermodulationLib/Overmodulation  OverModType=Flat top
      settings: LibrarySourceBlock=sps_lib/Power Electronics/Power Electronics Control/Overmodulation
  PLL & Measurements : Subsystem
  Pref : Constant  Value=0
  Pref1 : Constant  Value=300e3
  Rectifier : spsUniversalBridgeLib/Universal Bridge  Arms=3  SnubberResistance=0.1  SnubberCapacitance=0.1e-6  Device=Diodes  Ron=1e-3  Lon=0  ForwardVoltages="[  0.8  0.8  ]"  ForwardVoltage=.8  GTOparameters=[ 10e-6 , 20e-6 ]  IGBTparameters=[ 1e-6 , 2e-6 ]  Measurements=Device currents  Measurements_2=None  converterType=Rectifier
      settings: AttributesFormatString=\n
  Three-Level NPC Converter : spsThreeLevelNPCConverterLib/Three-Level NPC Converter  ModelType=Average model (Uref-controlled)  Ron=1e-3  Rs=1e6  Cs=inf  Vforward=[0,0]  Ron_Diode=1e-3  Rs_Diode=1e6  Cs_Diode=inf  Vf_Diode=1e-3  Rs_CurrentSource=inf  Ron_ACsource=1e-3
      settings: LibrarySourceBlock=|
      | sps_lib/Power Electronics/Three-Level
      | NPC Converter
  Unit Delay : UnitDelay  SampleTime=Ts_Control  HasFrameUpgradeWarning=on
  inv : spsThreePhaseVIMeasurementLib/Three-Phase V-I Measurement  VoltageMeasurement=phase-to-phase  SetLabelV=on  LabelV=Vinv  Vpu=off  VpuLL=off  CurrentMeasurement=no  SetLabelI=on  LabelI=Iload  Ipu=off  Pbase=1e3  Vbase=380  OutputType=Magnitude  PhasorSimulation=off  PSBequivalent=0
  wind generation : Subsystem
  A : PMIOPort  Side=Right
  B : PMIOPort  Port=2  Side=Right
  C_ : PMIOPort  Port=3  Side=Right
  wires:
  Overmodulation/1 -> [Uref]
  [Uref] -> Three-Level NPC Converter/1
  Mux/1 -> Battery Controller/1(PQref)
  Pref1/1 -> Mux/1  "Pref"
  Pref/1 -> Mux/2  "Qref"
  PLL & Measurements/3(IdIq_prim) -> Current Control/3(IdIq_meas)
  [Vabc_B1] -> PLL & Measurements/1(Vabc_prim)
  [Iabc_B1] -> PLL & Measurements/2(Iabc_prim)
  PLL & Measurements/2(VdVq_prim) -> Current Control/2(VdVq_meas)
  Battery Controller/1(Idq_ref) -> Current Control/4(IdIq_ref)
  PLL & Measurements/1(wt) -> Current Control/1(wt)
  Current Control/1(Uabc) -> Unit Delay/1
  Unit Delay/1 -> Overmodulation/1
  connections:
  B1/RConn1 -- A/RConn1
  B1/RConn2 -- B/RConn1
  B1/RConn3 -- C_/RConn1
  100 kVA 260V / 25 kV/LConn3 -- B1/LConn3
  100 kVA 260V / 25 kV/LConn2 -- B1/LConn2
  100 kVA 260V / 25 kV/LConn1 -- B1/LConn1
  DC Link/RConn3 -- Three-Level NPC Converter/RConn3
  DC Link/RConn2 -- Three-Level NPC Converter/RConn2
  DC Link/LConn2 -- Rectifier/RConn2
  DC Link/LConn1 -- Rectifier/RConn1
  Three-Level NPC Converter/RConn1 -- DC Link/RConn1
  "2 mH "/RConn3 -- 10 kvar/LConn3 -- 100 kVA 260V / 25 kV/RConn3
  "2 mH "/RConn2 -- 10 kvar/LConn2 -- 100 kVA 260V / 25 kV/RConn2
  10 kvar/LConn1 -- 100 kVA 260V / 25 kV/RConn1 -- "2 mH "/RConn1
  inv/LConn2 -- Three-Level NPC Converter/LConn2
  Rectifier/LConn2 -- wind generation/RConn2
  inv/LConn3 -- Three-Level NPC Converter/LConn3
  inv/RConn2 -- "2 mH "/LConn2
  inv/RConn3 -- "2 mH "/LConn3
  Rectifier/LConn1 -- wind generation/RConn1
  inv/LConn1 -- Three-Level NPC Converter/LConn1
  Rectifier/LConn3 -- wind generation/RConn3
  inv/RConn1 -- "2 mH "/LConn1

== system BATTERY_PV_IMPLEMENTATION/Controlled PV Array/PV Array ==
  note: Allows PV model to initialize
  T : Inport
  G : Inport  Port=2
  V_dc : Inport  Port=3
  I_dc : Inport  Port=4
  Controlled Current Source19 : spsControlledCurrentSourceLib/Controlled Current Source  Initialize=on  Source_Type=AC  Amplitude=0  Phase=0  Frequency=0  Measurements=None
  Delay : Delay  DelayLength=1  InitialCondition=1000
  Delay1 : Delay  DelayLength=1  InitialCondition=1200
  Display : Display
  I module : MATLABFcn  MATLABFcn=Np*u(2)-Np*u(1)*(exp((u(3)/(Ns)+Rs*u(4)/Np)/((Ns_cell*k*(u(5)+273.15)/q)*a))-1)-Np*((u(3)/(Ns)+Rs*u(4)/Np)/Rp)  OutputDimensions=1
  I0 : MATLABFcn  MATLABFcn=(Isc_n+KI*(u(1)-Tn))/(exp((Voc_n+KV*(u(1)-Tn))/((Ns_cell*k*(u(1)+273.15)/q)*a))-1);  OutputDimensions=1
  Ipv : MATLABFcn  MATLABFcn=(Ipv_n+KI*(u(1)-Tn))*(u(2)/Gn);  OutputDimensions=1
  Mux : Mux  Inputs=2
  Mux1 : Mux  Inputs=5
  Product17 : Product
  Saturation : Saturate  UpperLimit=10e6  LowerLimit=0.1
  Step16 : Step  Time=0.001  SampleTime=0
  PV+ : PMIOPort  Side=Right
  PV- : PMIOPort  Port=2  Side=Right
  wires:
  Mux1/1 -> I module/1
  G/1 -> Mux/2
  Mux/1 -> Ipv/1
  T/1 -> Mux1/5, Mux/1, I0/1
  Ipv/1 -> Mux1/2
  I0/1 -> Mux1/1
  Delay/1 -> Mux1/4
  I_dc/1 -> Delay/1
  Saturation/1 -> Product17/1
  Step16/1 -> Product17/2
  Product17/1 -> Controlled Current Source19/1
  Delay1/1 -> Mux1/3
  V_dc/1 -> Delay1/1
  I module/1 -> Display/1, Saturation/1
  connections:
  PV+/RConn1 -- Controlled Current Source19/RConn1
  Controlled Current Source19/LConn1 -- PV-/RConn1

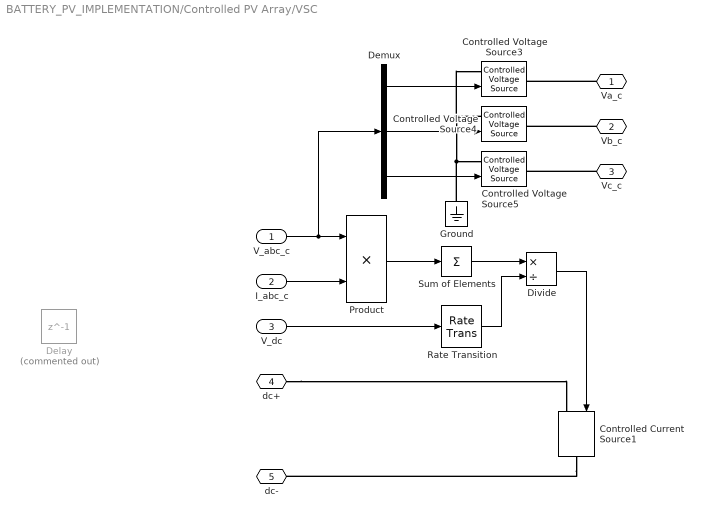
== system BATTERY_PV_IMPLEMENTATION/Controlled PV Array/VSC ==
  V_abc_c : Inport
  I_abc_c : Inport  Port=2
  V_dc : Inport  Port=3
  Controlled Current Source1 : spsControlledCurrentSourceLib/Controlled Current Source  Initialize=on  Source_Type=AC  Amplitude=0  Phase=0  Frequency=0  Measurements=None
  Controlled Voltage Source3 : spsControlledVoltageSourceLib/Controlled Voltage Source  Initialize=off  Source_Type=AC  Amplitude=0  Phase=0  Frequency=60  Measurements=None
  Controlled Voltage Source4 : spsControlledVoltageSourceLib/Controlled Voltage Source  Initialize=off  Source_Type=AC  Amplitude=0  Phase=0  Frequency=60  Measurements=None
  Controlled Voltage Source5 : spsControlledVoltageSourceLib/Controlled Voltage Source  Initialize=off  Source_Type=AC  Amplitude=0  Phase=0  Frequency=60  Measurements=None
  Delay : Delay  Commented=on  DelayLength=1  InitialCondition=1200
  Demux : Demux  Outputs=3
  Divide : Product  Inputs=*/  RndMeth=Zero  SaturateOnIntegerOverflow=on
  Ground : spsGroundLib/Ground  LConnTagsString=a
  Product : Product
  Rate Transition : RateTransition
  Sum of Elements : Sum  Inputs=+
  Va_c : PMIOPort  Side=Left
  Vb_c : PMIOPort  Port=2  Side=Left
  Vc_c : PMIOPort  Port=3  Side=Left
  dc+ : PMIOPort  Port=4  Side=Right
  dc- : PMIOPort  Port=5  Side=Right
  wires:
  Product/1 -> Sum of Elements/1
  I_abc_c/1 -> Product/2
  V_abc_c/1 -> Demux/1, Product/1
  Demux/2 -> Controlled Voltage Source4/1
  Demux/1 -> Controlled Voltage Source3/1
  Demux/3 -> Controlled Voltage Source5/1
  Sum of Elements/1 -> Divide/1
  Divide/1 -> Controlled Current Source1/1
  V_dc/1 -> Rate Transition/1
  Rate Transition/1 -> Divide/2
  connections:
  Vb_c/RConn1 -- Controlled Voltage Source4/RConn1
  Va_c/RConn1 -- Controlled Voltage Source3/RConn1
  Controlled Voltage Source4/LConn1 -- Controlled Voltage Source3/LConn1 -- Controlled Voltage Source5/LConn1 -- Ground/LConn1
  Vc_c/RConn1 -- Controlled Voltage Source5/RConn1
  Controlled Current Source1/RConn1 -- dc-/RConn1
  dc+/RConn1 -- Controlled Current Source1/LConn1

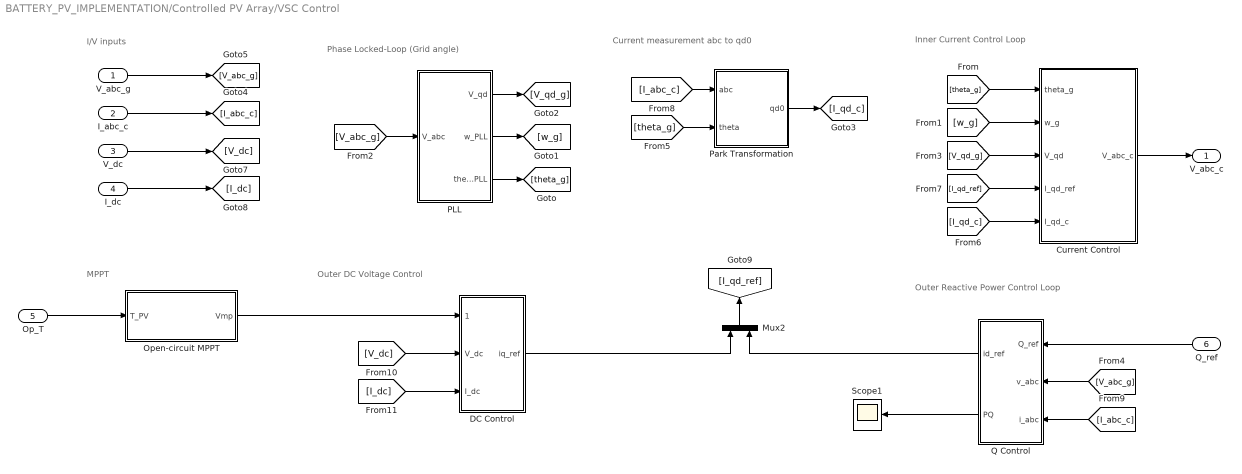
== system BATTERY_PV_IMPLEMENTATION/Controlled PV Array/VSC Control ==
  note: I/V inputs
  note: Phase Locked-Loop (Grid angle)
  note: Current measurement abc to qd0
  note: Inner Current Control Loop
  note: Outer Reactive Power Control Loop
  note: MPPT
  note: Outer DC Voltage Control
  V_abc_g : Inport
  I_abc_c : Inport  Port=2
  V_dc : Inport  Port=3
  I_dc : Inport  Port=4
  Op_T : Inport  Port=5
  Q_ref : Inport  Port=6
  Current Control : Subsystem
  DC Control : Subsystem
  Mux2 : Mux  Inputs=2
  Open-circuit MPPT : Subsystem
  PLL : Subsystem
  Park Transformation : Subsystem
  Q Control : Subsystem
  Scope1 : Scope
  V_abc_c : Outport
  wires:
  Park Transformation/1(qd0) -> [I_qd_c]
  [theta_g] -> Current Control/1(theta_g)
  PLL/3(theta_PLL) -> [theta_g]
  [I_qd_ref] -> Current Control/4(I_qd_ref)
  [theta_g] -> Park Transformation/2(theta)
  PLL/1(V_qd) -> [V_qd_g]
  PLL/2(w_PLL) -> [w_g]
  [w_g] -> Current Control/2(w_g)
  [V_qd_g] -> Current Control/3(V_qd)
  [I_qd_c] -> Current Control/5(I_qd_c)
  Current Control/1(V_abc_c) -> V_abc_c/1
  [V_abc_g] -> Q Control/2(v_abc)
  [I_abc_c] -> Q Control/3(i_abc)
  [V_dc] -> DC Control/2(V_dc)
  [I_dc] -> DC Control/3(I_dc)
  [I_abc_c] -> Park Transformation/1(abc)
  V_dc/1 -> [V_dc]
  I_abc_c/1 -> [I_abc_c]
  V_abc_g/1 -> [V_abc_g]
  I_dc/1 -> [I_dc]
  DC Control/1(iq_ref) -> Mux2/1
  Q Control/1(id_ref) -> Mux2/2
  Mux2/1 -> [I_qd_ref]
  Q_ref/1 -> Q Control/1(Q_ref)
  Op_T/1 -> Open-circuit MPPT/1(T_PV)
  Q Control/2(PQ) -> Scope1/1
  Open-circuit MPPT/1(Vmp) -> DC Control/1(V_dc_ref)
  [V_abc_g] -> PLL/1(V_abc)

== system BATTERY_PV_IMPLEMENTATION/Subsystem/Battery Controller ==
  m : Inport
  PQref : Inport  Port=2
  Compute PQ : Subsystem
  "P,Q Control " : Subsystem  TreatAsAtomicUnit=on
  to PU : Gain  Gain=1/Pnom
  Idq_ref : Outport  VectorParamsAs1DForOutWhenUnconnected=off
  wires:
  Compute PQ/1(PQm) -> "P,Q Control "/2(m)
  PQref/1 -> to PU/1
  m/1 -> Compute PQ/1(m)
  to PU/1 -> "P,Q Control "/1(PQref)
  "P,Q Control "/1(Idq_ref) -> Idq_ref/1

== system BATTERY_PV_IMPLEMENTATION/Subsystem/DC Link ==
  C1 : spsSeriesRLCBranchLib/Series RLC Branch  LConnTagsString=__new0  RConnTagsString=__new0  BranchType=C  Resistance=1.0  Inductance=1.0  SetiL0=off  InitialCurrent=0  Capacitance=Clink  Setx0=on  InitialVoltage=Vnom_dc/2  Measurements=None
  C2 : spsSeriesRLCBranchLib/Series RLC Branch  LConnTagsString=__new0  RConnTagsString=__new0  BranchType=C  Resistance=1e5  Inductance=1.0  SetiL0=off  InitialCurrent=0  Capacitance=Clink  Setx0=on  InitialVoltage=Vnom_dc/2  Measurements=None
  PV+ : PMIOPort  Side=Left
  PV-- : PMIOPort  Port=2  Side=Left
  Inv+ : PMIOPort  Port=3  Side=Right
  N : PMIOPort  Port=4  Side=Right
  Inv-- : PMIOPort  Port=5  Side=Right
  connections:
  C1/LConn1 -- PV+/RConn1 -- Inv+/RConn1
  C2/LConn1 -- N/RConn1 -- C1/RConn1
  C2/RConn1 -- PV--/RConn1 -- Inv--/RConn1

== system BATTERY_PV_IMPLEMENTATION/Subsystem/Grid Inverter ==
  note: Harmonic Filter
  Uref : Inport
  10 kvar : spsThreePhaseSeriesRLCLoadLib/Three-Phase Series RLC Load  LConnTagsString=A|B|C  Configuration=Delta  NominalVoltage=Vnom_sec  Vabc=[1e3 1e3 1e3]  Vabcp=[1e3 1e3 1e3]  NominalFrequency=Fnom  UnbalancedPower=off  ActivePower=Pc  InductivePower=0  CapacitivePower=Qc  Pabc=[10e3 9e3 11e3]  QLabc=[100 90 110]  QCabc=[100 90 110]  Pabcp=[10e3 9e3 11e3]  QLabcp=[100 90 110]  QCabcp=[100 90 110]  Measurements=None  LoadType=constant Z
  100 kVA 260V / 25 kV : spsThreePhaseTransformerTwoWindingsLib/Three-Phase Transformer (Two Windings)  Winding1Connection=Yg  Winding2Connection=Delta (D1)  CoreType=Three single-phase transformers  SetSaturation=off  Hysteresis=off  DataFile='hysteresis'  SetInitialFlux=off  Measurements=None  UNITS=pu  NominalPower=[Pnom Fnom ]  Winding1=[ Vnom_prim , Rxf/2 , Lxf/2 ]  Winding2=[ Vnom_sec , Rxf/2 , Lxf/2 ]  Rm=200  Lm=200  L0=0.5  Saturation=[ 0,0 ; 0.0024,1.2 ; 1.0,1.52 ]  InitialFluxes=[ 0.8 , -0.8 , 0.7 ]  BreakLoop=off  DiscreteSolver=Trapezoidal iterative  DataType=off  TransfoNumber=0
  B1 : spsThreePhaseVIMeasurementLib/Three-Phase V-I Measurement  VoltageMeasurement=phase-to-ground  SetLabelV=off  LabelV=Vabc_B1  Vpu=off  VpuLL=off  CurrentMeasurement=yes  SetLabelI=off  LabelI=Iabc_B1  Ipu=off  Pbase=100e6  Vbase=500e3  OutputType=Magnitude  PhasorSimulation=off  PSBequivalent=0
  Bus Creator : BusCreator  Inputs=2
  Ground : Ground
  L : spsThreePhaseSeriesRLCBranchLib/Three-Phase Series RLC Branch  LConnTagsString=A|B|C  RConnTagsString=A|B|C  BranchType=RL  Resistance=Rchoke*Zbase  Inductance=Lchoke*Zbase/(2*pi*Fnom)  Capacitance=inf  Measurements=None
  Three-Level NPC Converter : spsThreeLevelNPCConverterLib/Three-Level NPC Converter  ModelType=Average model (Uref-controlled)  Ron=1e-3  Rs=1e6  Cs=inf  Vforward=[0,0]  Ron_Diode=1e-3  Rs_Diode=1e6  Cs_Diode=inf  Vf_Diode=1e-3  Rs_CurrentSource=inf  Ron_ACsource=1e-3
      settings: LibrarySourceBlock=|
      | sps_lib/Power Electronics/Three-Level
      | NPC Converter
  Inv+ : PMIOPort  Side=Left
  N : PMIOPort  Port=2  Side=Left
  Inv-- : PMIOPort  Port=3  Side=Left
  A : PMIOPort  Port=4  Side=Right
  B : PMIOPort  Port=5  Side=Right
  C : PMIOPort  Port=6  Side=Right
  m : Outport  VectorParamsAs1DForOutWhenUnconnected=off
  wires:
  Ground/1 -> Three-Level NPC Converter/2
  Bus Creator/1 -> m/1
  B1/2 -> Bus Creator/2  "Iabc"
  B1/1 -> Bus Creator/1  "Vabc"
  Uref/1 -> Three-Level NPC Converter/1
  connections:
  N/RConn1 -- Three-Level NPC Converter/RConn2
  Three-Level NPC Converter/LConn3 -- L/LConn3
  Three-Level NPC Converter/LConn2 -- L/LConn2
  Three-Level NPC Converter/LConn1 -- L/LConn1
  100 kVA 260V / 25 kV/LConn1 -- B1/LConn1
  100 kVA 260V / 25 kV/LConn2 -- B1/LConn2
  100 kVA 260V / 25 kV/LConn3 -- B1/LConn3
  10 kvar/LConn2 -- 100 kVA 260V / 25 kV/RConn2 -- L/RConn2
  10 kvar/LConn3 -- 100 kVA 260V / 25 kV/RConn3 -- L/RConn3
  Three-Level NPC Converter/RConn3 -- Inv--/RConn1
  Three-Level NPC Converter/RConn1 -- Inv+/RConn1
  L/RConn1 -- 100 kVA 260V / 25 kV/RConn1 -- 10 kvar/LConn1
  B1/RConn1 -- A/RConn1
  B1/RConn2 -- B/RConn1
  B1/RConn3 -- C/RConn1

== system BATTERY_PV_IMPLEMENTATION/Subsystem/Inverter Control ==
  Vabc_prim : Inport  PortDimensions=3
  Iabc_prim : Inport  Port=2  PortDimensions=3
  Idq_ref : Inport  Port=3
  Current Control : Subsystem  TreatAsAtomicUnit=on
  Overmodulation : spsOvermodulationLib/Overmodulation  OverModType=Flat top
      settings: LibrarySourceBlock=sps_lib/Power Electronics/Power Electronics Control/Overmodulation
  PLL & Measurements : Subsystem
  Unit Delay : UnitDelay  SampleTime=Ts_Control  HasFrameUpgradeWarning=on
  Uref : Outport  VectorParamsAs1DForOutWhenUnconnected=off
  wires:
  Vabc_prim/1 -> PLL & Measurements/1(Vabc_prim)
  Iabc_prim/1 -> PLL & Measurements/2(Iabc_prim)
  PLL & Measurements/3(IdIq_prim) -> Current Control/3(IdIq_meas)
  PLL & Measurements/2(VdVq_prim) -> Current Control/2(VdVq_meas)
  PLL & Measurements/1(wt) -> Current Control/1(wt)
  Idq_ref/1 -> Current Control/4(IdIq_ref)
  Current Control/1(Uabc) -> Unit Delay/1
  Overmodulation/1 -> Uref/1
  Unit Delay/1 -> Overmodulation/1

== system BATTERY_PV_IMPLEMENTATION/Subsystem2/Battery Controller ==
  PQref : Inport
  Compute PQ : Subsystem
  "P,Q Control " : Subsystem  TreatAsAtomicUnit=on
  to PU : Gain  Gain=1/Pnom
  Idq_ref : Outport  VectorParamsAs1DForOutWhenUnconnected=off
  wires:
  [Iabc_B1] -> Compute PQ/2(IABC)
  [Vabc_B1] -> Compute PQ/1(VABC)
  "P,Q Control "/1(Idq_ref) -> Idq_ref/1
  to PU/1 -> "P,Q Control "/1(PQref)
  PQref/1 -> to PU/1
  Compute PQ/1(PQm) -> "P,Q Control "/2(m)

== system BATTERY_PV_IMPLEMENTATION/Subsystem2/Current Control ==
  wt : Inport
  VdVq_meas : Inport  Port=2  PortDimensions=2
  IdIq_meas : Inport  Port=3  PortDimensions=2
  IdIq_ref : Inport  Port=4  PortDimensions=2
  Current Regulator : Subsystem
  Uabc_ref Generation max (m) = 1 : Subsystem
  Uabc : Outport  VectorParamsAs1DForOutWhenUnconnected=off
  wires:
  Uabc_ref Generation max (m) = 1/1(Uabc_ref) -> Uabc/1
  IdIq_ref/1 -> Current Regulator/3(IdIq_ref)
  IdIq_meas/1 -> Current Regulator/2(IdIq_meas)
  VdVq_meas/1 -> Current Regulator/1(VdVq_meas)
  Current Regulator/1(VdVq_conv) -> Uabc_ref Generation max (m) = 1/2(VdVq_conv)
  wt/1 -> Uabc_ref Generation max (m) = 1/1(wt)

== system BATTERY_PV_IMPLEMENTATION/Subsystem2/DC Link ==
  C1 : spsSeriesRLCBranchLib/Series RLC Branch  LConnTagsString=__new0  RConnTagsString=__new0  BranchType=C  Resistance=1.0  Inductance=1.0  SetiL0=off  InitialCurrent=0  Capacitance=Clink  Setx0=on  InitialVoltage=Vnom_dc/2  Measurements=None
  C2 : spsSeriesRLCBranchLib/Series RLC Branch  LConnTagsString=__new0  RConnTagsString=__new0  BranchType=C  Resistance=1e5  Inductance=1.0  SetiL0=off  InitialCurrent=0  Capacitance=Clink  Setx0=on  InitialVoltage=Vnom_dc/2  Measurements=None
  PV+ : PMIOPort  Side=Left
  PV-- : PMIOPort  Port=2  Side=Left
  Inv+ : PMIOPort  Port=3  Side=Right
  N : PMIOPort  Port=4  Side=Right
  Inv-- : PMIOPort  Port=5  Side=Right
  connections:
  Inv--/RConn1 -- PV--/RConn1 -- C2/RConn1
  C1/RConn1 -- N/RConn1 -- C2/LConn1
  Inv+/RConn1 -- PV+/RConn1 -- C1/LConn1

== system BATTERY_PV_IMPLEMENTATION/Subsystem2/PLL & Measurements ==
  note: PLL & Measurements
      | ===================
  Vabc_prim : Inport
  Iabc_prim : Inport  Port=2
  PLL (3ph) : spsPLL3phLib/PLL (3ph)  Fmin=45  Par_Init="[-0.57  Fnom]"  ParK=[180, 3200, 1]  TcD=Ts_Control  MaxRateChangeFreq=12  FilterCutOffFreq=25  Ts=Ts_Control  AGC=on
  Selector1 : Selector  InputPortWidth=3  IndexOptions=Index vector (dialog)  Indices=[1 2]  OutputSizes=1
  Selector2 : Selector  InputPortWidth=3  IndexOptions=Index vector (dialog)  Indices=[1 2]  OutputSizes=1
  Terminator : Terminator
  V->pu : Gain  Gain=1/(Vnom_prim*sqrt(2)/sqrt(3))  SaturateOnIntegerOverflow=on  OutDataTypeStr=Inherit: Same as input  ParamDataTypeStr=Inherit: Same as input
  V->pu1 : Gain  Gain=Vnom_prim*sqrt(3)/Pnom/sqrt(2)  SaturateOnIntegerOverflow=on  OutDataTypeStr=Inherit: Same as input  ParamDataTypeStr=Inherit: Same as input
  abc to dq0 : spsabctodq0Lib/abc to dq0  Alignment=90 degrees behind phase A axis
  abc to dq1 : spsabctodq0Lib/abc to dq0  Alignment=90 degrees behind phase A axis
  wt : Outport  VectorParamsAs1DForOutWhenUnconnected=off
  VdVq_prim : Outport  Port=2  VectorParamsAs1DForOutWhenUnconnected=off
  IdIq_prim : Outport  Port=3  VectorParamsAs1DForOutWhenUnconnected=off
  wires:
  V->pu1/1 -> abc to dq1/1
  V->pu/1 -> PLL (3ph)/1, abc to dq0/1
  abc to dq1/1 -> Selector1/1
  Vabc_prim/1 -> V->pu/1
  Iabc_prim/1 -> V->pu1/1
  abc to dq0/1 -> Selector2/1
  Selector2/1 -> VdVq_prim/1
  Selector1/1 -> IdIq_prim/1
  PLL (3ph)/2 -> wt/1, abc to dq1/2, abc to dq0/2
  PLL (3ph)/1 -> Terminator/1
